simulink model "siasun_config_casadi_VS_lsj_robot_16a"  (R2020a)
settings: Solver=FixedStepAuto  StartTime=0.0  StopTime=inf  FixedStep=0.001  RelTol=1e-3  EnableMultiTasking=on
libraries: Robot_ToolBox x20
(part 6 of 6)

== matlab function siasun_config_casadi_VS_lsj_robot_16a/Robot1/Set Control/Torque/Set Mode/Not ==
  data: in input; out output
function out = fcn(in)

if in == 0
    out = 1;
else
    out = 0;
end

end

== matlab function siasun_config_casadi_VS_lsj_robot_16a/Robot1/Set Control/Torque/power and start ==
  data: input_power input; output output; input_start input
function output  = fcn(input_power, input_start)

if (input_power == 1) && (input_start == 1)
    output = 1;
else
    output = 0;
end

end

== matlab function siasun_config_casadi_VS_lsj_robot_16a/Robot1/Set Control/Velocity/Set Mode/Not ==
  data: in input; out output
function out = fcn(in)

if in == 0
    out = 1;
else
    out = 0;
end

end

== matlab function siasun_config_casadi_VS_lsj_robot_16a/Robot1/Set Control/Velocity/power and start ==
  data: input_power input; output output; input_start input
function output  = fcn(input_power, input_start)

if (input_power == 1) && (input_start == 1)
    output = 1;
else
    output = 0;
end

end

== matlab function siasun_config_casadi_VS_lsj_robot_16a/Robot1/Time/MATLAB Function ==
  data: set input; t_out output; t_in input
function t_out = timer(set, t_in)

persistent flag;
if isempty(flag)
    flag = 0;
end

if set == 1
    t_out = t_in + 0.001;
else
    t_out = 0;
end

end

== matlab function siasun_config_casadi_VS_lsj_robot_16a/Cartesian_planning_angle/DH-IK4 ==
  data: angle1 input; t input; Radian output; angle2 input
function Radian  = read(angle1,t,angle2)
if t <= 5
    Radian = angle2;
else
    Radian = angle1;
end
end

== matlab function siasun_config_casadi_VS_lsj_robot_16a/Cartesian_planning_angle/sampling_switch ==
  data: out output; t input
function out   = sampling_switch( t)
if (t>10&&t<=15)
    out=int32(1);
else
    out=int32(0); 
end
end

== matlab function siasun_config_casadi_VS_lsj_robot_16a/Cartesian_planning_angle/三阶曲线规划1/一关节/3_planning1 ==
  data: state output; plan3_A output; g_vs parameter; g_ve parameter; S input; tf input; tf output
function [state, plan3_A,tf] =planning3( g_vs, g_ve,S,tf)
% 三次多项式算法主程序
% vs初始速度m/min,ve末速度m/min,S总位移m,
% 基础插补规划函数
% 三次多项式速度规划
    a0 = 0 ;
    a1 = g_vs ;
    a2 = 3*S/tf^2 - 2* g_vs/tf - g_ve/tf;
    a3 = -2*S/tf^3 - (g_vs+g_ve)/tf^2;
    state = 1;
    plan3_A = [a0 a1 a2 a3];
    tf =tf ;

end

== matlab function siasun_config_casadi_VS_lsj_robot_16a/Cartesian_planning_angle/三阶曲线规划1/一关节/Interpolation3 ==
  data: state output; Enable input; Y output; plan3_A input; tf input; t input
function [state, Y]  = Interpolate3(Enable,plan3_A,tf,t)
%% input
a0 = plan3_A(1);
a1 = plan3_A(2);
a2 = plan3_A(3);
a3 = plan3_A(4);
Y = 0;
%% output
if Enable == 1
    if t <=tf
    Y = a0 + a1*t + a2*t^2 + a3*t^3; 
    state =1;
    else
    Y = a0 + a1*tf + a2*tf^2 + a3*tf^3;
    state = 1;
    end
else 
    Y = 0;
    state = 0;
end
end

== matlab function siasun_config_casadi_VS_lsj_robot_16a/Cartesian_planning_angle/三阶曲线规划1/三关节/3_planning1 ==
  data: state output; plan3_A output; g_vs parameter; g_ve parameter; S input; tf input; tf output
function [state, plan3_A,tf] =planning3( g_vs, g_ve,S,tf)
% 三次多项式算法主程序
% vs初始速度m/min,ve末速度m/min,S总位移m,
% 基础插补规划函数
% 三次多项式速度规划
    a0 = 0 ;
    a1 = g_vs ;
    a2 = 3*S/tf^2 - 2* g_vs/tf - g_ve/tf;
    a3 = -2*S/tf^3 - (g_vs+g_ve)/tf^2;
    state = 1;
    plan3_A = [a0 a1 a2 a3];
    tf =tf ;

end

== matlab function siasun_config_casadi_VS_lsj_robot_16a/Cartesian_planning_angle/三阶曲线规划1/二关节/3_planning1 ==
  data: state output; plan3_A output; g_vs parameter; g_ve parameter; S input; tf input; tf output
function [state, plan3_A,tf] =planning3( g_vs, g_ve,S,tf)
% 三次多项式算法主程序
% vs初始速度m/min,ve末速度m/min,S总位移m,
% 基础插补规划函数
% 三次多项式速度规划
    a0 = 0 ;
    a1 = g_vs ;
    a2 = 3*S/tf^2 - 2* g_vs/tf - g_ve/tf;
    a3 = -2*S/tf^3 - (g_vs+g_ve)/tf^2;
    state = 1;
    plan3_A = [a0 a1 a2 a3];
    tf =tf ;

end

== matlab function siasun_config_casadi_VS_lsj_robot_16a/Cartesian_planning_angle/三阶曲线规划1/二关节/Interpolation3 ==
  data: state output; Enable input; Y output; plan3_A input; tf input; t input
function [state, Y]  = Interpolate3(Enable,plan3_A,tf,t)
%% input
a0 = plan3_A(1);
a1 = plan3_A(2);
a2 = plan3_A(3);
a3 = plan3_A(4);
Y = 0;
%% output
if Enable == 1
    if t <=tf
    Y = a0 + a1*t + a2*t^2 + a3*t^3; 
    state =1;
    else
    Y = a0 + a1*tf + a2*tf^2 + a3*tf^3;
    state = 1;
    end
else 
    Y = 0;
    state = 0;
end
end

== matlab function siasun_config_casadi_VS_lsj_robot_16a/Cartesian_planning_angle/三阶曲线规划1/五关节/3_planning1 ==
  data: state output; plan3_A output; g_vs parameter; g_ve parameter; S input; tf input; tf output
function [state, plan3_A,tf] =planning3( g_vs, g_ve,S,tf)
% 三次多项式算法主程序
% vs初始速度m/min,ve末速度m/min,S总位移m,
% 基础插补规划函数
% 三次多项式速度规划
    a0 = 0 ;
    a1 = g_vs ;
    a2 = 3*S/tf^2 - 2* g_vs/tf - g_ve/tf;
    a3 = -2*S/tf^3 - (g_vs+g_ve)/tf^2;
    state = 1;
    plan3_A = [a0 a1 a2 a3];
    tf =tf ;

end

== matlab function siasun_config_casadi_VS_lsj_robot_16a/Cartesian_planning_angle/三阶曲线规划1/三关节/Interpolation3 ==
  data: state output; Enable input; Y output; plan3_A input; tf input; t input
function [state, Y]  = Interpolate3(Enable,plan3_A,tf,t)
%% input
a0 = plan3_A(1);
a1 = plan3_A(2);
a2 = plan3_A(3);
a3 = plan3_A(4);
Y = 0;
%% output
if Enable == 1
    if t <=tf
    Y = a0 + a1*t + a2*t^2 + a3*t^3; 
    state =1;
    else
    Y = a0 + a1*tf + a2*tf^2 + a3*tf^3;
    state = 1;
    end
else 
    Y = 0;
    state = 0;
end
end

== matlab function siasun_config_casadi_VS_lsj_robot_16a/Cartesian_planning_angle/三阶曲线规划1/五关节/Interpolation3 ==
  data: state output; Enable input; Y output; plan3_A input; tf input; t input
function [state, Y]  = Interpolate3(Enable,plan3_A,tf,t)
%% input
a0 = plan3_A(1);
a1 = plan3_A(2);
a2 = plan3_A(3);
a3 = plan3_A(4);
Y = 0;
%% output
if Enable == 1
    if t <=tf
    Y = a0 + a1*t + a2*t^2 + a3*t^3; 
    state =1;
    else
    Y = a0 + a1*tf + a2*tf^2 + a3*tf^3;
    state = 1;
    end
else 
    Y = 0;
    state = 0;
end
end

== matlab function siasun_config_casadi_VS_lsj_robot_16a/Cartesian_planning_angle/三阶曲线规划1/六关节/3_planning1 ==
  data: state output; plan3_A output; g_vs parameter; g_ve parameter; S input; tf input; tf output
function [state, plan3_A,tf] =planning3( g_vs, g_ve,S,tf)
% 三次多项式算法主程序
% vs初始速度m/min,ve末速度m/min,S总位移m,
% 基础插补规划函数
% 三次多项式速度规划
    a0 = 0 ;
    a1 = g_vs ;
    a2 = 3*S/tf^2 - 2* g_vs/tf - g_ve/tf;
    a3 = -2*S/tf^3 - (g_vs+g_ve)/tf^2;
    state = 1;
    plan3_A = [a0 a1 a2 a3];
    tf =tf ;

end

== matlab function siasun_config_casadi_VS_lsj_robot_16a/Cartesian_planning_angle/三阶曲线规划1/六关节/Interpolation3 ==
  data: state output; Enable input; Y output; plan3_A input; tf input; t input
function [state, Y]  = Interpolate3(Enable,plan3_A,tf,t)
%% input
a0 = plan3_A(1);
a1 = plan3_A(2);
a2 = plan3_A(3);
a3 = plan3_A(4);
Y = 0;
%% output
if Enable == 1
    if t <=tf
    Y = a0 + a1*t + a2*t^2 + a3*t^3; 
    state =1;
    else
    Y = a0 + a1*tf + a2*tf^2 + a3*tf^3;
    state = 1;
    end
else 
    Y = 0;
    state = 0;
end
end

== matlab function siasun_config_casadi_VS_lsj_robot_16a/Cartesian_planning_angle/三阶曲线规划1/四关节/3_planning1 ==
  data: state output; plan3_A output; g_vs parameter; g_ve parameter; S input; tf input; tf output
function [state, plan3_A,tf] =planning3( g_vs, g_ve,S,tf)
% 三次多项式算法主程序
% vs初始速度m/min,ve末速度m/min,S总位移m,
% 基础插补规划函数
% 三次多项式速度规划
    a0 = 0 ;
    a1 = g_vs ;
    a2 = 3*S/tf^2 - 2* g_vs/tf - g_ve/tf;
    a3 = -2*S/tf^3 - (g_vs+g_ve)/tf^2;
    state = 1;
    plan3_A = [a0 a1 a2 a3];
    tf =tf ;

end

== matlab function siasun_config_casadi_VS_lsj_robot_16a/Cartesian_planning_angle/三阶曲线规划1/四关节/Interpolation3 ==
  data: state output; Enable input; Y output; plan3_A input; tf input; t input
function [state, Y]  = Interpolate3(Enable,plan3_A,tf,t)
%% input
a0 = plan3_A(1);
a1 = plan3_A(2);
a2 = plan3_A(3);
a3 = plan3_A(4);
Y = 0;
%% output
if Enable == 1
    if t <=tf
    Y = a0 + a1*t + a2*t^2 + a3*t^3; 
    state =1;
    else
    Y = a0 + a1*tf + a2*tf^2 + a3*tf^3;
    state = 1;
    end
else 
    Y = 0;
    state = 0;
end
end

== matlab function siasun_config_casadi_VS_lsj_robot_16a/Robot1/Limit and Logic/Joint Limit ==
  data: mode input; power_in input; set_angle input; read_angle input; target_angle input; joint_limit input; power_out output
function power_out = fcn(mode, power_in, set_angle, read_angle, target_angle, joint_limit)

if mode == 1
    for i = 1 : 6
        if (set_angle(i) < joint_limit(2*i-1)) || (set_angle(i) > joint_limit(2*i))
            power_out = 0;
            break;
        else
            power_out = power_in;
            continue;
        end
    end
    
else
    for i = 1 : 6
        if (read_angle(i) < joint_limit(2*i-1)) ...
                || (read_angle(i)> joint_limit(2*i)) ...
                || (target_angle(i) < joint_limit(2*i-1)) ...
                || (target_angle(i)> joint_limit(2*i))
            power_out = 0;
            break;
        else
            power_out = power_in;
            continue;
        end
    end
end
    
end
